simulink model "InvkinTest"  (R2019b)
settings: Solver=VariableStepAuto  StartTime=0.0  StopTime=10  RelTol=1e-3
values from neighbouring files (symbols this model uses):
  R = SerialLink(L, 'name', '210F', 'comment', 'six DOF', 'manufacturer', 'FANUC')    [Model_210F.m]    (also in Model_210F_old.m)
undefined symbols (not defined in the file or in its folder): transl, trotx
libraries: roblocks x8
settings Model: Creator=Karl  LastModifiedBy=Karl

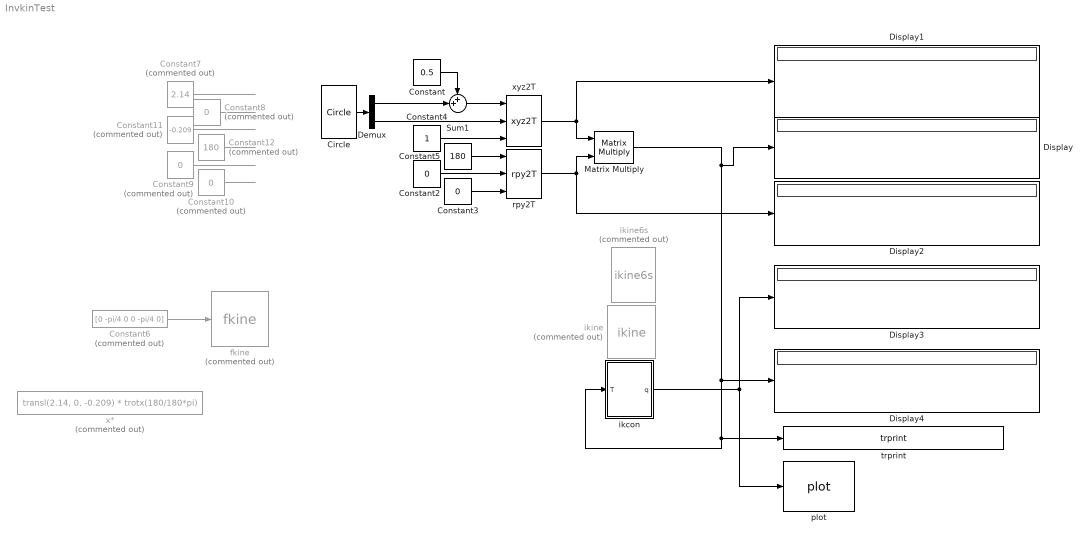
== system InvkinTest ==
  Circle : roblocks/Toolbox/Circle  radius=0.5  freq=0.2
  Constant : Constant  Value=0.5
  Constant10 : Constant  Commented=on  Value=0
  Constant11 : Constant  Commented=on  Value=-0.209
  Constant12 : Constant  Commented=on  Value=180
  Constant2 : Constant  Value=0
  Constant3 : Constant  Value=0
  Constant4 : Constant
  Constant5 : Constant  Value=180
  Constant6 : Constant  Commented=on  Value=[0 -pi/4 0 0 -pi/4 0]
  Constant7 : Constant  Commented=on  Value=2.14
  Constant8 : Constant  Commented=on  Value=0
  Constant9 : Constant  Commented=on  Value=0
  Demux : Demux  Outputs=2
  Display{,1..4} (5 alike) : Display
  Matrix Multiply : Product  Multiplication=Matrix(*)
  Sum1 : Sum  Inputs=++|
  fkine : roblocks/Arm/fkine  Commented=on  robot=R
  ikcon : Subsystem  mask{robot=R}
      mask prompts: robot "Robot object"
      mask help: Inverse kinematics for 6-axis spherical robot
      mask Help:
      | Compute joint coordinates for robot given end-effector pose.
      | 
      | 
      | <b>Parameters::</b>
      | 
      | Robot (SerialLink class)  The N-axis robot object for computing forward kinematics.
      | Configuration             Configuration string comprised of 'lrudnf'
      | 
      | <b>Inputs::</b>
      | 
      | T (4x4) the pose of the end effector as a homogeneous transformation
      | 
      | 
      | <b>Outputs::</b>
      | 
      | q (1xN) joint coordinates
      | 
      | <b>Notes::</b>
      | 
      | - A wrapper for the Toolbox method ikine6s().
  ikine : roblocks/Arm/ikine  Commented=on  robot=R  q0=qz  M=[1 1 1 1 1 1]  pinv=off  options={}
  ikine6s : roblocks/Arm/ikine6s  Commented=on  robot=R  conf='u'
  plot : roblocks/Arm/plot  robot=R  fps=5  holdplot=on
  rpy2T : roblocks/Toolbox/rpy2T  sequence=ZYX  degrees=on
  trprint : roblocks/Toolbox/trprint  options={'bingo'}
  x* : Constant  Commented=on  Value=transl(2.14, 0, -0.209) * trotx(180/180*pi)
  xyz2T : roblocks/Toolbox/xyz2T
  wires:
  Constant5/1 -> rpy2T/1
  Constant4/1 -> xyz2T/3
  Constant3/1 -> rpy2T/3
  Constant2/1 -> rpy2T/2
  xyz2T/1 -> Matrix Multiply/1, Display1/1
  rpy2T/1 -> Matrix Multiply/2, Display2/1
  ikcon/1(q) -> plot/1, Display3/1
  Constant6/1 -> fkine/1
  Matrix Multiply/1 -> ikcon/1(T), trprint/1, Display4/1, Display/1
  Constant12/1 -> ?
  Constant9/1 -> ?
  Constant8/1 -> ?
  Constant7/1 -> ?
  Constant11/1 -> ?
  Constant10/1 -> ?
  Circle/1 -> Demux/1
  Demux/1 -> Sum1/2
  Demux/2 -> xyz2T/2
  Sum1/1 -> xyz2T/1
  Constant/1 -> Sum1/1

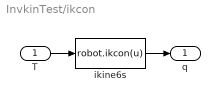
== system InvkinTest/ikcon ==
  T : Inport
  ikine6s : MATLABFcn  MATLABFcn=robot.ikcon(u)  OutputDimensions=6
  q : Outport  VectorParamsAs1DForOutWhenUnconnected=off
  wires:
  T/1 -> ikine6s/1
  ikine6s/1 -> q/1
